simulink subsystem "PowerGain"  (R2023a)
settings: Solver=VariableStepAuto  StartTime=0.0  StopTime=10.0  RelTol=1e-3
undefined symbols (not defined in the file): gain_pw, max_output_voltage
settings Model: Creator=ycheb  LastModifiedBy=ycheb

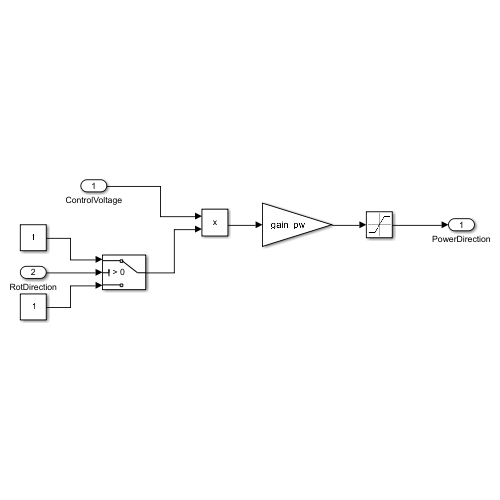
[thumbnail: Simulink's stored preview of the top-level diagram]
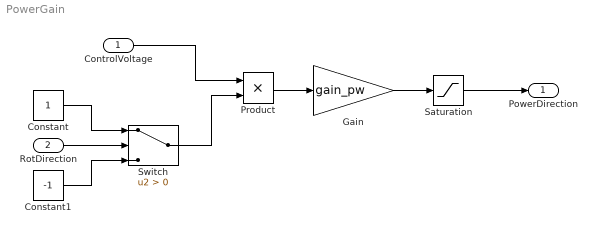
== system PowerGain ==
  ControlVoltage : Inport
  RotDirection : Inport  Port=2  OutDataTypeStr=boolean
  Constant : Constant
  Constant1 : Constant  Value=-1
  Gain : Gain  Gain=gain_pw
  Product : Product
  Saturation : Saturate  UpperLimit=max_output_voltage  LowerLimit=-max_output_voltage
  Switch : Switch  Criteria=u2 > Threshold  SaturateOnIntegerOverflow=off  InputSameDT=off
  PowerDirection : Outport
  wires:
  Saturation/1 -> PowerDirection/1
  Gain/1 -> Saturation/1
  Product/1 -> Gain/1
  ControlVoltage/1 -> Product/1
  RotDirection/1 -> Switch/2
  Constant1/1 -> Switch/3
  Constant/1 -> Switch/1
  Switch/1 -> Product/2
